simulink model "DTNS_KAISIM"  (R2022a)
settings: Solver=FixedStepDiscrete  StartTime=0.0  StopTime=200  FixedStep=0.04  RelTol=1e-3
PreLoadFcn:
  | listing = dir;
  | if (contains([listing .name], 'DTNS_KAISIM.slx'))
  |     addpath('./TCAF', './TRN', './FTG', './DYN', './FLCC', './GPS', './RALT', './INS', './MAP', './AGR');
  | else
  | 
  | end
  | 
  | load('BUS_STRUCTURE_DYN.mat');
  | load('BUS_STRUCTURE_FLCC.mat');
  | load('BUS_STRUCTURE_RALT.mat');
  | load('BUS_STRUCTURE_INS.mat');
  | load('BUS_STRUCTURE_GPS.mat');
  | load('BUS_STRUCTURE_SENSOR_INPUT.mat');
  | load('BusStructureTRN.mat');
  | load('BusStructureWTPG.mat');
  | load('BusStructureDTF.mat');
  | load('BusStructureGCAWS.mat');
  | load('BusStructureCR.mat');
  | load('BusStructureHR.mat');
  | load('BusStructureLOSR.mat');
  | 
  | clear logsout
InitFcn:
  | listing = dir;
  | if (contains([listing .name], 'DTNS_KAISIM.slx'))
  |     addpath('./TCAF', './TRN', './FTG', './DYN', './FLCC', './GPS', './RALT', './INS', './MAP', './AGR');
  | else
  | 
  | end
  | 
  | load('BUS_STRUCTURE_DYN.mat');
  | load('BUS_STRUCTURE_FLCC.mat');
  | load('BUS_STRUCTURE_RALT.mat');
  | load('BUS_STRUCTURE_INS.mat');
  | load('BUS_STRUCTURE_GPS.mat');
  | load('BUS_STRUCTURE_SENSOR_INPUT.mat');
  | load('BusStructureTRN.mat');
  | load('BusStructureWTPG.mat');
  | load('BusStructureDTF.mat');
  | load('BusStructureGCAWS.mat');
  | load('BusStructureCR.mat');
  | load('BusStructureHR.mat');
  | load('BusStructureLOSR.mat');
  | 
  | clear logsout
(part 1 of 2)
settings Model: Creator=ASCL  LastModifiedBy=halbu
settings SolverCC: PositivePriorityOrder=on
settings DataIOCC: ExternalInput=TCAF_WHOLESIMScenario.getElement('IN_TPF_WCPSIM_STICK'),TCAF_WHOLESIMScenario.getElement('IN_TPF_WCPSIM_FLIGHT_CMD'),TCAF_WHOLESIMScenario.getElement('IN_DTFIn'),TCAF_WHOLESIMScenario.getElement('IN_GCAWSIn')  SaveOutput=off  DSMLogging=off  ReturnWorkspaceOutputs=off
settings OptimizationCC: BlockReduction=off  DefaultParameterBehavior=Inlined  UseDivisionForNetSlopeComputation=on  GainParamInheritBuiltInType=on  UseFloatMulNetSlope=on  ExpressionFolding=off  PassReuseOutputArgsAs=Individual arguments  ZeroExternalMemoryAtStartup=off  ZeroInternalMemoryAtStartup=off  EfficientFloat2IntCast=on  LifeSpan=inf  OptimizeBlockOrder=speed  DifferentSizesBufferReuse=on  EfficientTunableParamExpr=on
settings DebuggingCC: SignalInfNanChecking=warning  ReadBeforeWriteMsg=EnableAllAsError  WriteAfterWriteMsg=EnableAllAsError  WriteAfterReadMsg=EnableAllAsError  IntegerOverflowMsg=error  ParameterTunabilityLossMsg=error  UniqueDataStoreMsg=error  AssertControl=DisableAll  NonBusSignalsTreatedAsBus=error  SFInvalidInputDataAccessInChartInitDiag=error  SFTransitionOutsideNaturalParentDiag=error  SFUnreachableExecutionPathDiag=error  SFUndirectedBroadcastEventsDiag=error  IntegerSaturationMsg=error
settings HardwareCC: ProdBitPerPointer=32  ProdBitPerSizeT=32  ProdBitPerPtrDiffT=32  ProdLargestAtomicInteger=Long  ProdLargestAtomicFloat=Double  ProdEndianess=BigEndian  ProdWordSize=32  ProdLongLongMode=on  ProdHWDeviceType=Freescale->MPC83xx
settings ModelReferenceCC: ModelReferenceNumInstancesAllowed=Single
settings SFSimCC: SimCustomHeaderCode="#include \"MAP.h\""  SimUserSources=MAP.c  SimUserLibraries=WS2_32.LIB  CompileTimeRecursionLimit=0  EnableRuntimeRecursion=off  MATLABDynamicMemAlloc=off
settings RTWCC: SystemTargetFile=ert.tlc  TemplateMakefile=ert_default_tmf  GenerateReport=on  RTWUseSimCustomCode=on  CustomHeaderCode="#include \"MAP.h\""  CustomSource=MAP.c  CustomLibrary=WS2_32.LIB  BuildConfiguration=Faster Runs  IncludeHyperlinkInReport=on  LaunchReport=on  GenerateTraceInfo=on  GenerateTraceReport=on  GenerateTraceReportSl=on  GenerateTraceReportSf=on  GenerateTraceReportEml=on
settings CodeAppCC: ForceParamTrailComments=on  IgnoreCustomStorageClasses=off  OperatorAnnotations=on  SimulinkDataObjDesc=on  SFDataObjDesc=on  MATLABFcnDesc=on  InsertBlockDesc=on  StateflowObjectComments=on  MATLABSourceComments=on  EnableCustomComments=on  InlinedPrmAccess=Macros  ReqsInCode=on
settings ERTTargetCC: TargetLangStandard=C99 (ISO)  UtilityFuncGeneration=Shared location  GenerateSampleERTMain=on  IncludeMdlTerminateFcn=off  CombineSignalStateStructs=on  SuppressErrorStatus=on  SupportAbsoluteTime=off  SupportNonFinite=off  SupportComplex=off  ParenthesesLevel=Standards  CastingMode=Standards  GenerateSharedConstants=off  InlinedParameterPlacement=NonHierarchical  ERTCustomFileTemplate=example_file_process.tlc  RateTransitionBlockCode=Function  PreserveIfCondition=on  ConvertIfToSwitch=off  EnableSignedLeftShifts=off  EnableSignedRightShifts=off

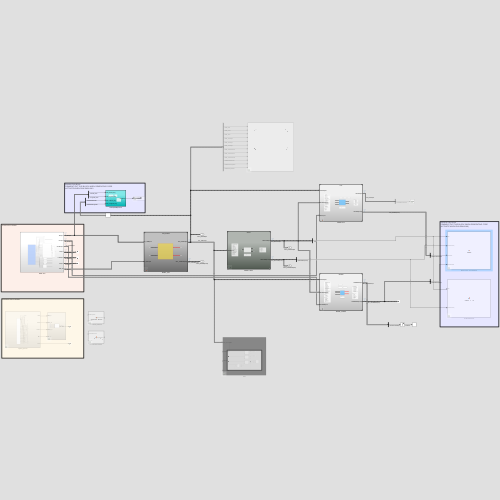
[thumbnail: Simulink's stored preview of the top-level diagram]
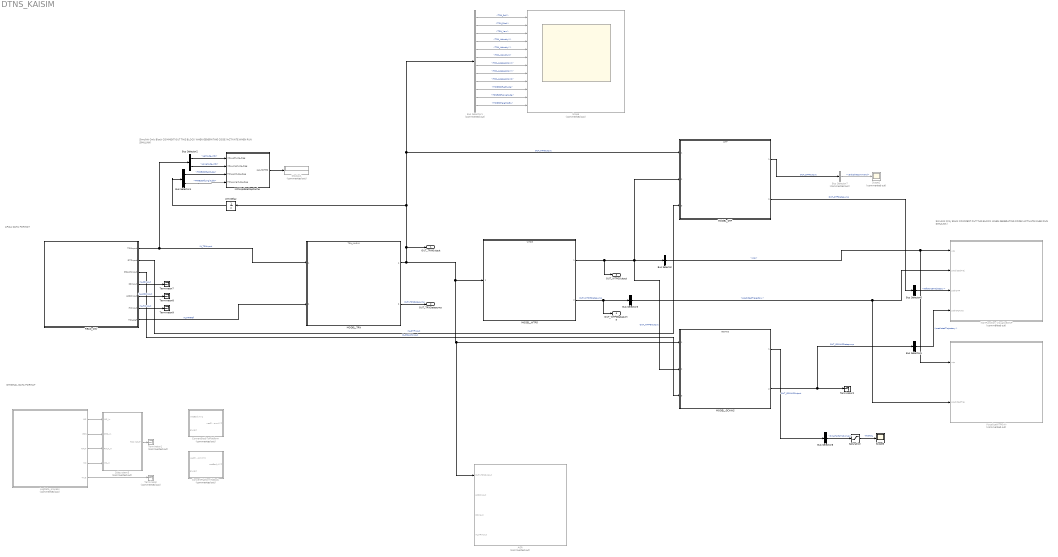
== system DTNS_KAISIM ==
  note: APIAA DATA FORMAT
  note: ORIGINAL DATA FORMAT
  note: Simulink Only Block
      | COMMENT OUT THIS BLOCK WHEN GENERATING CODE
      | (ACTIVATE WHEN RUN SIMULINK)
  note: Simulink Only Block
      | COMMENT OUT THIS BLOCK WHEN GENERATING CODE
      | (ACTIVATE WHEN RUN SIMULINK)
  AGR : Subsystem  Commented=on
  Bus Selector : BusSelector  OutputSignals=wtp
  Bus Selector1 : BusSelector  Commented=on  OutputSignals=TRN_Roll,TRN_Pitch,TRN_Yaw,TRN_VelocityX,TRN_VelocityY,TRN_VelocityZ,TRN_AccelerationX,TRN_AccelerationY,TRN_AccelerationZ,TRNEstOfLatitude,TRNEstOfLongitude,TRNEstHeightAGL
  Bus Selector2 : BusSelector  OutputSignals=Latitude_INS,Longitude_INS
  Bus Selector3 : BusSelector  OutputSignals=predictedTrajectory
  Bus Selector4 : BusSelector  OutputSignals=TRNEstOfLatitude,TRNEstOfLongitude
  Bus Selector5 : BusSelector  OutputSignals=predictedTrajectory
  Bus Selector6 : BusSelector  OutputSignals=referenceTrajectory
  Bus Selector7 : BusSelector  Commented=on  OutputSignals=verticalGCommand
  Bus Selector8 : BusSelector  OutputSignals=timeToGoToPullUp
  ConvertBodyToPlatform : MATLAB Function  Commented=on  TreatAsAtomicUnit=on
  ConvertPlatformToBody : MATLAB Function  Commented=on  TreatAsAtomicUnit=on
  Display1 : Display  Commented=on
  InitNUpdateMapCache : Subsystem  TreatAsAtomicUnit=on
  LogData_process : Subsystem  Commented=on
  MATFunction_VisualizeWCP : MATLAB Function  Commented=on  TreatAsAtomicUnit=on
  MODEL_DTF : ModelReference  ModelNameDialog=DTF.slx  SimulationMode=Normal  ModelReferenceVersion=1.428
  MODEL_GCAWS : ModelReference  ModelNameDialog=GCAWS.slx  SimulationMode=Normal  ModelReferenceVersion=1.774
  MODEL_TRN : ModelReference  ModelNameDialog=TRN_KAISIM.slx  SimulationMode=Normal  ModelReferenceVersion=2.352
  MODEL_WTPG : ModelReference  ModelNameDialog=WTPG.slx  SimulationMode=Normal  ModelReferenceVersion=1.377
  READ_CSV : Subsystem
  Saturation : Saturate  UpperLimit=5.0  LowerLimit=0.0
  Scope : Scope  Commented=on  NumInputPorts=12
  Scope1 : Scope  Commented=on
  Scope3 : Scope
  Subsystem3 : Subsystem  Commented=on
  Terminator : Terminator  Commented=on
  Terminator1 : Terminator  Commented=on
  Terminator{2,7..9} (4 alike) : Terminator
  Unit Delay : UnitDelay  SampleTime=-1  HasFrameUpgradeWarning=on
  VisualizeWTPOnly : MATLAB Function  Commented=on  TreatAsAtomicUnit=on
  OUT_TRNOutput : Outport  OutDataTypeStr=Bus: TRNOutput  BusOutputAsStruct=on
  OUT_TRNDatapump : Outport  Port=2  OutDataTypeStr=Bus: TRNDatapump
  OUT_WTPGOutput : Outport  Port=3  OutDataTypeStr=Bus: WTPGOutput
  OUT_WTPGDatapump : Outport  Port=4  OutDataTypeStr=Bus: WTPGDatapump
  wires:
  Bus Selector7/1 -> Scope1/1  "<verticalGCommand>"
  Bus Selector6/1 -> MATFunction_VisualizeWCP/3(pathDTF)  "<referenceTrajectory>"
  Bus Selector1/4 -> Scope/4  "<TRN_VelocityX>"
  MODEL_DTF/2 -> Bus Selector6/1  "OUT_DTFDatapump"
  Bus Selector5/1 -> MATFunction_VisualizeWCP/4(pathGCAWS)  "<predictedTrajectory>"
  Bus Selector1/5 -> Scope/5  "<TRN_VelocityY>"
  Bus Selector1/7 -> Scope/7  "<TRN_AccelerationX>"
  Bus Selector1/8 -> Scope/8  "<TRN_AccelerationY>"
  MODEL_WTPG/1 -> OUT_WTPGOutput/1, MODEL_GCAWS/2, MODEL_DTF/2, Bus Selector/1  "OUT_WTPGOutput"
  Bus Selector1/9 -> Scope/9  "<TRN_AccelerationZ>"
  Bus Selector1/12 -> Scope/12  "<TRNEstHeightAGL>"
  Bus Selector1/11 -> Scope/11  "<TRNEstOfLongitude>"
  MODEL_TRN/1 -> Unit Delay/1, Bus Selector1/1, MODEL_DTF/1, OUT_TRNOutput/1, AGR/1(OUT_TRNOutput), MODEL_GCAWS/1, MODEL_WTPG/1  "OUT_TRNOutput"
  MODEL_WTPG/2 -> OUT_WTPGDatapump/1, Bus Selector3/1  "OUT_WTPGDatapump"
  Bus Selector1/3 -> Scope/3  "<TRN_Yaw>"
  MODEL_GCAWS/2 -> Bus Selector5/1, Terminator2/1  "OUT_GCAWSDatapump"
  Bus Selector1/10 -> Scope/10  "<TRNEstOfLatitude>"
  MODEL_TRN/2 -> OUT_TRNDatapump/1  "OUT_TRNDatapump"
  MODEL_GCAWS/1 -> Bus Selector8/1  "OUT_GCAWSOutput"
  Bus Selector1/6 -> Scope/6  "<TRN_VelocityZ>"
  Bus Selector3/1 -> VisualizeWTPOnly/2(predictedTraj), MATFunction_VisualizeWCP/2(predictedTraj)  "<predictedTrajectory>"
  READ_CSV/1(TRNInput) -> Bus Selector2/1, MODEL_TRN/1  "IN_TRNInput"
  Bus Selector/1 -> VisualizeWTPOnly/1(wtp), MATFunction_VisualizeWCP/1(wtp)  "<wtp>"
  Bus Selector1/1 -> Scope/1  "<TRN_Roll>"
  MODEL_DTF/1 -> Bus Selector7/1  "OUT_DTFOutput"
  Bus Selector1/2 -> Scope/2  "<TRN_Pitch>"
  Bus Selector8/1 -> Saturation/1  "<timeToGoToPullUp>"
  Saturation/1 -> Scope3/1  "TTGTPU"
  READ_CSV/2(DTFInput) -> MODEL_DTF/3  "IN_DTFInput"
  READ_CSV/3(GCAWSInput) -> MODEL_GCAWS/3  "IN_GCAWSInput"
  Bus Selector2/1 -> InitNUpdateMapCache/1(INS_Latitude_Deg)  "<Latitude_INS>"
  Bus Selector2/2 -> InitNUpdateMapCache/2(INS_Longitude_Deg)  "<Longitude_INS>"
  READ_CSV/5(LOSRInput) -> Terminator8/1  "IN_LOSRInput"
  READ_CSV/4(CRInput) -> Terminator7/1  "IN_CRInput"
  InitNUpdateMapCache/1(resultDTED) -> Display1/1
  READ_CSV/6(HRInput) -> Terminator9/1  "IN_HRInput"
  LogData_process/1(INS) -> Subsystem3/1(INS_In)
  LogData_process/2(GPS) -> Subsystem3/2(GPS_In)
  LogData_process/3(RALT) -> Subsystem3/3(RALT_In)
  LogData_process/4(MC) -> Subsystem3/4(MC_In)
  LogData_process/5(True) -> Terminator/1
  Subsystem3/1(TRN INPUT) -> Terminator1/1
  READ_CSV/7(TRN_Ref) -> MODEL_TRN/2  "IN_TRNRef"
  Bus Selector4/1 -> InitNUpdateMapCache/3(TRN_Latitude_Deg)  "<TRNEstOfLatitude>"
  Bus Selector4/2 -> InitNUpdateMapCache/4(TRN_Longitude_Deg)  "<TRNEstOfLongitude>"
  Unit Delay/1 -> Bus Selector4/1

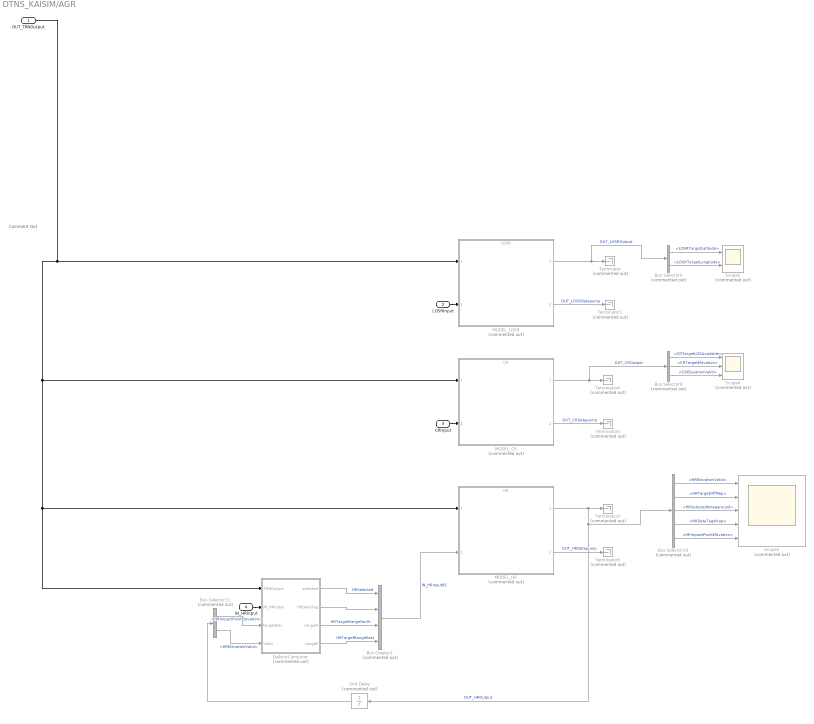
== system DTNS_KAISIM/AGR ==
  note: Comment Out
  OUT_TRNOutput : Inport
  LOSRInput : Inport  Port=2
  CRInput : Inport  Port=3
  IN_HRInput : Inport  Port=4
  BallisticComputer : MATLAB Function  Commented=on  TreatAsAtomicUnit=on
  Bus Creator3 : BusCreator  Commented=on  Inputs=4  OutDataTypeStr=Bus: HRInput  NonVirtualBus=on
      settings: InheritFromInputs=off
  Bus Selector10 : BusSelector  Commented=on  OutputSignals=HRElevationValid,HRTargetOffMap,HRSelectedWraparound,HRDataTagWrap,HRImpactPointElevation
  Bus Selector11 : BusSelector  Commented=on  OutputSignals=HRImpactPointElevation,HRElevationValid
  Bus Selector4 : BusSelector  Commented=on  OutputSignals=LOSRTargetLatitude,LOSRTargetLongitude
  Bus Selector9 : BusSelector  Commented=on  OutputSignals=CRTargetLOSAvailable,CRTargetElevation,CRElevationValid
  MODEL_CR : ModelReference  Commented=on  ModelNameDialog=CR.slx  SimulationMode=Normal  ModelReferenceVersion=1.236
  MODEL_HR : ModelReference  Commented=on  ModelNameDialog=HR.slx  SimulationMode=Normal  ModelReferenceVersion=1.371
  MODEL_LOSR : ModelReference  Commented=on  ModelNameDialog=LOSR.slx  SimulationMode=Normal  ModelReferenceVersion=1.331
  Scope2 : Scope  Commented=on  NumInputPorts=2
  Scope4 : Scope  Commented=on  NumInputPorts=3
  Scope5 : Scope  Commented=on  NumInputPorts=5
  Terminator{,1,3..6} (6 alike) : Terminator  Commented=on
  Unit Delay : UnitDelay  Commented=on  SampleTime=-1  HasFrameUpgradeWarning=on
  wires:
  MODEL_LOSR/1 -> Bus Selector4/1, Terminator/1  "OUT_LOSROutput"
  Bus Selector10/3 -> Scope5/3  "<HRSelectedWraparound>"
  MODEL_HR/1 -> Unit Delay/1, Bus Selector10/1, Terminator3/1  "OUT_HROutput"
  Bus Selector9/2 -> Scope4/2  "<CRTargetElevation>"
  BallisticComputer/2(HRDataTag) -> Bus Creator3/2
  Bus Creator3/1 -> MODEL_HR/2  "IN_HRInputBC"
  Bus Selector9/1 -> Scope4/1  "<CRTargetLOSAvailable>"
  MODEL_HR/2 -> Terminator6/1  "OUT_HRDatapump"
  Bus Selector10/1 -> Scope5/1  "<HRElevationValid>"
  MODEL_CR/1 -> Bus Selector9/1, Terminator4/1  "OUT_CROutput"
  Bus Selector4/2 -> Scope2/2  "<LOSRTargetLongitude>"
  OUT_TRNOutput/1 -> BallisticComputer/1(TRNOutput), MODEL_HR/1, MODEL_CR/1, MODEL_LOSR/1
  Bus Selector10/2 -> Scope5/2  "<HRTargetOffMap>"
  LOSRInput/1 -> MODEL_LOSR/2
  MODEL_CR/2 -> Terminator5/1  "OUT_CRDatapump"
  Bus Selector10/5 -> Scope5/5  "<HRImpactPointElevation>"
  MODEL_LOSR/2 -> Terminator1/1  "OUT_LOSRDatapump"
  BallisticComputer/4(rangeE) -> Bus Creator3/4  "HRTargetRangeEast"
  Bus Selector4/1 -> Scope2/1  "<LOSRTargetLatitude>"
  Bus Selector10/4 -> Scope5/4  "<HRDataTagWrap>"
  Unit Delay/1 -> Bus Selector11/1
  IN_HRInput/1 -> BallisticComputer/2(IN_HRInput)
  BallisticComputer/3(rangeN) -> Bus Creator3/3  "HRTargetRangeNorth"
  Bus Selector11/2 -> BallisticComputer/4(Valid)  "<HRElevationValid>"
  Bus Selector9/3 -> Scope4/3  "<CRElevationValid>"
  BallisticComputer/1(selected) -> Bus Creator3/1  "HRSelected"
  Bus Selector11/1 -> BallisticComputer/3(targetElev)  "<HRImpactPointElevation>"
  CRInput/1 -> MODEL_CR/2

== system DTNS_KAISIM/InitNUpdateMapCache ==
  INS_Latitude_Deg : Inport  OutDataTypeStr=double
  INS_Longitude_Deg : Inport  Port=2  OutDataTypeStr=double
  TRN_Latitude_Deg : Inport  Port=3
  TRN_Longitude_Deg : Inport  Port=4
  If : If  NumInputs=2  IfExpression=(u1 == 0)  ShowElse=off
  InitializeMAP : MATLAB Function  TreatAsAtomicUnit=on
  UpdateCache : Subsystem  TreatAsAtomicUnit=on
  resultDTED : Outport  VectorParamsAs1DForOutWhenUnconnected=off
  wires:
  INS_Longitude_Deg/1 -> UpdateCache/2(INS_Longitude_Deg)
  UpdateCache/1(result) -> resultDTED/1
  InitializeMAP/1(successDTED) -> If/1
  INS_Latitude_Deg/1 -> UpdateCache/1(INS_Latitude_Deg)
  InitializeMAP/2(successDVOF) -> If/2
  If/1 -> UpdateCache/Action
  TRN_Latitude_Deg/1 -> UpdateCache/3(TRN_Latitude_Deg)
  TRN_Longitude_Deg/1 -> UpdateCache/4(TRN_Longitude_Deg)

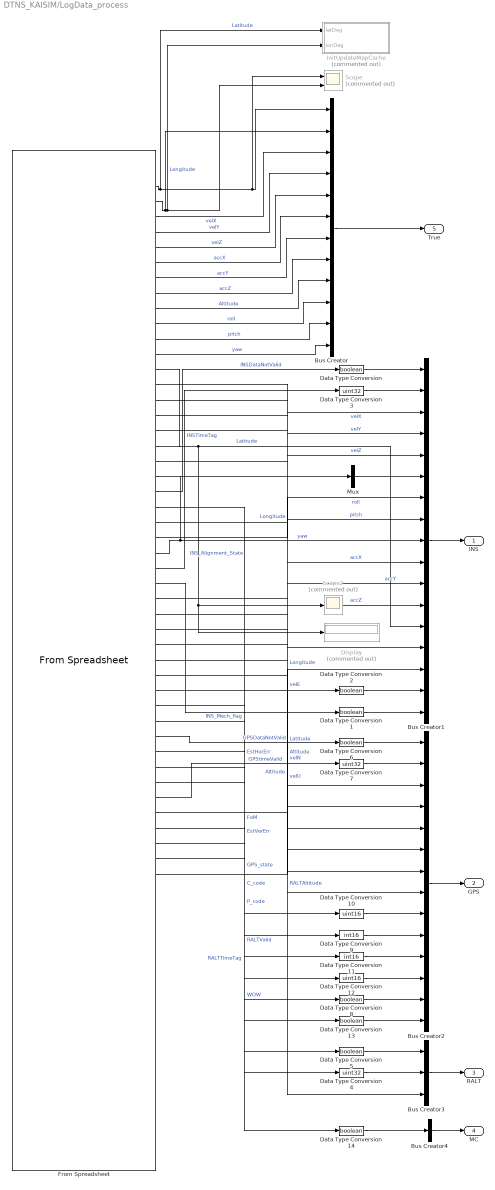
== system DTNS_KAISIM/LogData_process ==
  Bus Creator : BusCreator  Inputs=12  OutDataTypeStr=Bus: TRN_Ref
      settings: InheritFromInputs=off
  Bus Creator1 : BusCreator  Inputs=17  OutDataTypeStr=Bus: TRN_INS
      settings: InheritFromInputs=off
  Bus Creator2 : BusCreator  Inputs=14  OutDataTypeStr=Bus: TRN_GPS
      settings: InheritFromInputs=off
  Bus Creator3 : BusCreator  Inputs=3  OutDataTypeStr=Bus: TRN_RALT
      settings: InheritFromInputs=off
  Bus Creator4 : BusCreator  Inputs=1  OutDataTypeStr=Bus: TRN_MC
      settings: InheritFromInputs=off
  Data Type Conversion{,1..2,5..6,8,13..14} (8 alike) : DataTypeConversion  OutDataTypeStr=boolean  SaturateOnIntegerOverflow=off  RndMeth=Floor
  Data Type Conversion10 : DataTypeConversion  OutDataTypeStr=uint16  SaturateOnIntegerOverflow=off  RndMeth=Floor
  Data Type Conversion11 : DataTypeConversion  OutDataTypeStr=int16  SaturateOnIntegerOverflow=off  RndMeth=Floor
  Data Type Conversion12 : DataTypeConversion  OutDataTypeStr=uint16  SaturateOnIntegerOverflow=off  RndMeth=Floor
  Data Type Conversion3 : DataTypeConversion  OutDataTypeStr=uint32  SaturateOnIntegerOverflow=off  RndMeth=Floor
  Data Type Conversion4 : DataTypeConversion  OutDataTypeStr=uint32  SaturateOnIntegerOverflow=off  RndMeth=Floor
  Data Type Conversion7 : DataTypeConversion  OutDataTypeStr=uint32  SaturateOnIntegerOverflow=off  RndMeth=Floor
  Data Type Conversion9 : DataTypeConversion  OutDataTypeStr=int16  SaturateOnIntegerOverflow=off  RndMeth=Floor
  Display : Display  Commented=on
  From Spreadsheet : FromSpreadsheet  FileName=KAI_input.csv  SheetName=KAI_input  TreatFirstColumnAs=Data  SampleTime=-1
  InitUpdateMapCache : Subsystem  Commented=on  TreatAsAtomicUnit=on
  Mux : Mux  Inputs=1
  Scope : Scope  Commented=on  NumInputPorts=2
  Scope2 : Scope  Commented=on
  INS : Outport  OutDataTypeStr=Bus: TRN_INS
  GPS : Outport  Port=2  OutDataTypeStr=Bus: TRN_GPS
  RALT : Outport  Port=3  OutDataTypeStr=Bus: TRN_RALT
  MC : Outport  Port=4  OutDataTypeStr=Bus: TRN_MC
  True : Outport  Port=5  OutDataTypeStr=Bus: TRN_Ref
  wires:
  From Spreadsheet/23 -> Data Type Conversion2/1  "INS_Alignment_State"
  From Spreadsheet/22 -> Data Type Conversion/1  "INSDataNotValid"
  From Spreadsheet/21 -> Bus Creator1/12  "accZ"
  From Spreadsheet/20 -> Bus Creator1/11  "accY"
  Bus Creator/1 -> True/1
  From Spreadsheet/27 -> Data Type Conversion3/1  "INSTimeTag"
  From Spreadsheet/25 -> Bus Creator1/8  "pitch"
  From Spreadsheet/24 -> Bus Creator1/7  "roll"
  From Spreadsheet/4 -> Bus Creator/3  "velX"
  From Spreadsheet/5 -> Bus Creator/4  "velY"
  From Spreadsheet/6 -> Bus Creator/5  "velZ"
  From Spreadsheet/7 -> Bus Creator/6  "accX"
  From Spreadsheet/8 -> Bus Creator/7  "accY"
  From Spreadsheet/9 -> Bus Creator/8  "accZ"
  From Spreadsheet/10 -> Bus Creator/9  "Altitude"
  From Spreadsheet/11 -> Bus Creator/10  "roll"
  From Spreadsheet/12 -> Bus Creator/11  "pitch"
  From Spreadsheet/13 -> Bus Creator/12  "yaw"
  From Spreadsheet/15 -> Bus Creator1/14  "Longitude"
  From Spreadsheet/19 -> Bus Creator1/10  "accX"
  From Spreadsheet/16 -> Bus Creator1/3  "velX"
  From Spreadsheet/17 -> Bus Creator1/4  "velY"
  From Spreadsheet/18 -> Bus Creator1/5  "velZ"
  Bus Creator1/1 -> INS/1
  From Spreadsheet/36 -> Data Type Conversion11/1  "EstVerErr"
  From Spreadsheet/37 -> Data Type Conversion10/1  "FoM"
  From Spreadsheet/38 -> Data Type Conversion6/1  "GPSDataNotValid"
  From Spreadsheet/39 -> Data Type Conversion12/1  "GPS_state"
  Bus Creator3/1 -> RALT/1
  Bus Creator2/1 -> GPS/1
  From Spreadsheet/28 -> Data Type Conversion1/1  "INS_Mech_flag"
  From Spreadsheet/29 -> Bus Creator2/3  "Latitude"
  From Spreadsheet/30 -> Bus Creator2/4  "Longitude"
  From Spreadsheet/31 -> Bus Creator2/6  "velE"
  From Spreadsheet/34 -> Bus Creator2/5  "Altitude"
  From Spreadsheet/35 -> Data Type Conversion9/1  "EstHorErr"
  From Spreadsheet/33 -> Bus Creator2/8  "velU"
  From Spreadsheet/32 -> Bus Creator2/7  "velN"
  Bus Creator4/1 -> MC/1
  Data Type Conversion/1 -> Bus Creator1/1
  Data Type Conversion3/1 -> Bus Creator1/2
  Data Type Conversion2/1 -> Bus Creator1/16
  Data Type Conversion5/1 -> Bus Creator3/1
  Data Type Conversion4/1 -> Bus Creator3/2
  Data Type Conversion7/1 -> Bus Creator2/2
  Data Type Conversion6/1 -> Bus Creator2/1
  Data Type Conversion1/1 -> Bus Creator1/17
  Data Type Conversion10/1 -> Bus Creator2/9
  Data Type Conversion8/1 -> Bus Creator2/13
  Data Type Conversion9/1 -> Bus Creator2/10
  From Spreadsheet/46 -> Data Type Conversion14/1  "WOW"
  From Spreadsheet/45 -> Data Type Conversion4/1  "RALTTimeTag"
  From Spreadsheet/44 -> Data Type Conversion5/1  "RALTValid"
  From Spreadsheet/47 -> Bus Creator1/15  "Altitude"
  Data Type Conversion14/1 -> Bus Creator4/1
  Data Type Conversion13/1 -> Bus Creator2/14
  From Spreadsheet/40 -> Data Type Conversion8/1  "C_code"
  From Spreadsheet/41 -> Data Type Conversion13/1  "P_code"
  From Spreadsheet/42 -> Data Type Conversion7/1  "GPStimeValid"
  From Spreadsheet/43 -> Bus Creator3/3  "RALTAltitude"
  Data Type Conversion12/1 -> Bus Creator2/12
  Data Type Conversion11/1 -> Bus Creator2/11
  Mux/1 -> Bus Creator1/6
  From Spreadsheet/2 -> Scope/1, Bus Creator/1, InitUpdateMapCache/1(latDeg)  "Latitude"
  From Spreadsheet/3 -> InitUpdateMapCache/2(lonDeg), Scope/2, Bus Creator/2  "Longitude"
  From Spreadsheet/26 -> Mux/1, Bus Creator1/9  "yaw"
  From Spreadsheet/14 -> Display/1, Scope2/1, Bus Creator1/13  "Latitude"

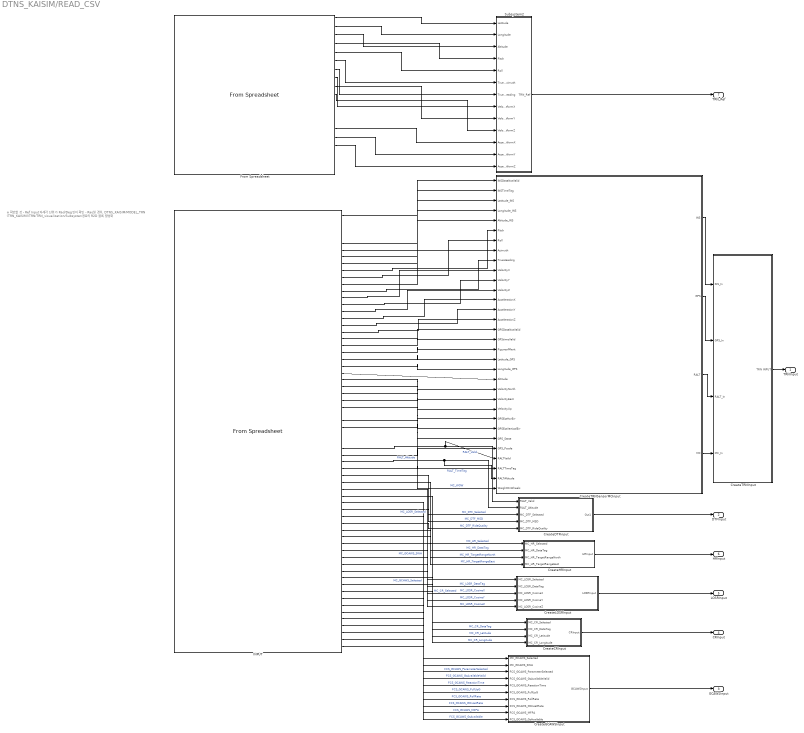
== system DTNS_KAISIM/READ_CSV ==
  note: ※ 확인할 것
      | - Ref Input 자세각 단위가 Rad/Deg 인지 확인
      | - Rad일 경우, DTNS_KAISIM/MODEL_TRN (TRN_KAISIM)/TRN/TRN_visualization/Subsystem2 경로의 R2D 블록 활성화
  CreateCRInput : Subsystem
  CreateDTFInput : Subsystem
  CreateGCAWSInput : Subsystem
  CreateHRInput : Subsystem
  CreateLOSRInput : Subsystem
  CreateTRNInput : Subsystem
  CreateTRNSensorMCInput : Subsystem
  From Spreadsheet : FromSpreadsheet  FileName=C:\Users\halbu\Documents\GitHub\DTNS\data\test_TRUE.csv  SheetName=test_TRUE  OutDataTypeStr=double  SampleTime=0.04  ExtrapolationBeforeFirstDataPoint=Hold first value  InterpolationWithinTimeRange=Zero order hold  ExtrapolationAfterLastDataPoint=Hold last value
  INPUT : FromSpreadsheet  FileName=C:\Users\halbu\Documents\GitHub\DTNS\data\test_INPUT.csv  SheetName=test_INPUT  OutDataTypeStr=double  SampleTime=0.04  ExtrapolationBeforeFirstDataPoint=Hold first value  InterpolationWithinTimeRange=Zero order hold  ExtrapolationAfterLastDataPoint=Hold last value
  Subsystem2 : Subsystem
  TRNInput : Outport  OutDataTypeStr=Bus: TRNInput
  DTFInput : Outport  Port=2  OutDataTypeStr=Bus: DTFInput
  GCAWSInput : Outport  Port=3  OutDataTypeStr=Bus: GCAWSInput
  CRInput : Outport  Port=4  OutDataTypeStr=Bus: CRInput
  LOSRInput : Outport  Port=5  OutDataTypeStr=Bus: LOSRInput
  HRInput : Outport  Port=6  OutDataTypeStr=Bus: HRInput
  TRN_Ref : Outport  Port=7  OutDataTypeStr=Bus: TRN_Ref
  wires:
  Subsystem2/1(TRN_Ref) -> TRN_Ref/1
  INPUT/7 -> CreateTRNSensorMCInput/4(Longitude_INS)
  INPUT/6 -> CreateTRNSensorMCInput/3(Latitude_INS)
  INPUT/5 -> CreateTRNSensorMCInput/2(INSTimeTag)
  INPUT/14 -> CreateTRNSensorMCInput/11(VelocityY)
  INPUT/10 -> CreateTRNSensorMCInput/7(Roll)
  INPUT/22 -> CreateTRNSensorMCInput/19(Latitude_GPS)
  INPUT/11 -> CreateTRNSensorMCInput/8(Azimuth)
  INPUT/23 -> CreateTRNSensorMCInput/20(Longitude_GPS)
  INPUT/19 -> CreateTRNSensorMCInput/16(GPSDataNotValid)
  INPUT/13 -> CreateTRNSensorMCInput/10(VelocityX)
  INPUT/9 -> CreateTRNSensorMCInput/6(Pitch)
  INPUT/17 -> CreateTRNSensorMCInput/14(AccelerationY)
  CreateTRNSensorMCInput/2(GPS) -> CreateTRNInput/2(GPS_In)
  INPUT/21 -> CreateTRNSensorMCInput/18(FigureofMerit)
  CreateTRNSensorMCInput/1(INS) -> CreateTRNInput/1(INS_In)
  INPUT/57 -> CreateGCAWSInput/3(FCS_GCAWS_ParameterSelected)  "FCS_GCAWS_ParameterSelected"
  INPUT/61 -> CreateGCAWSInput/7(FCS_GCAWS_RollRate)  "FCS_GCAWS_RollRate"
  INPUT/58 -> CreateGCAWSInput/4(FCS_GCAWS_GsAvailableValid)  "FCS_GCAWS_GsAvailableValid"
  INPUT/62 -> CreateGCAWSInput/8(FCS_GCAWS_GOnsetRate)  "FCS_GCAWS_GOnsetRate"
  INPUT/59 -> CreateGCAWSInput/5(FCS_GCAWS_ReactionTime)  "FCS_GCAWS_ReactionTime"
  INPUT/63 -> CreateGCAWSInput/9(FCS_GCAWS_MFPA)  "FCS_GCAWS_MFPA"
  CreateGCAWSInput/1(GCAWSInput) -> GCAWSInput/1
  INPUT/60 -> CreateGCAWSInput/6(FCS_GCAWS_PullUpG)  "FCS_GCAWS_PullUpG"
  INPUT/64 -> CreateGCAWSInput/10(FCS_GCAWS_GsAvailable)  "FCS_GCAWS_GsAvailable"
  INPUT/56 -> CreateCRInput/4(MC_CR_Longitude)  "MC_CR_Longitude"
  CreateCRInput/1(CRInput) -> CRInput/1
  CreateLOSRInput/1(LOSRInput) -> LOSRInput/1
  INPUT/43 -> CreateGCAWSInput/1(MC_GCAWS_Selected)  "MC_GCAWS_Selected"
  INPUT/55 -> CreateCRInput/3(MC_CR_Latitude)  "MC_CR_Latitude"
  INPUT/51 -> CreateLOSRInput/3(MC_LOSR_CosineX)  "MC_LOSR_CosineX"
  INPUT/47 -> CreateHRInput/2(MC_HR_DataTag)  "MC_HR_DataTag"
  INPUT/45 -> CreateGCAWSInput/2(MC_GCAWS_SWH)  "MC_GCAWS_SWH"
  INPUT/41 -> CreateLOSRInput/1(MC_LOSR_Selected)  "MC_LOSR_Selected"
  INPUT/53 -> CreateLOSRInput/5(MC_LOSR_CosineZ)  "MC_LOSR_CosineZ"
  INPUT/49 -> CreateHRInput/4(MC_HR_TargetRangeEast)  "MC_HR_TargetRangeEast"
  CreateHRInput/1(HRInput) -> HRInput/1
  INPUT/52 -> CreateLOSRInput/4(MC_LOSR_CosineY)  "MC_LOSR_CosineY"
  INPUT/40 -> CreateHRInput/1(MC_HR_Selected)  "MC_HR_Selected"
  INPUT/48 -> CreateHRInput/3(MC_HR_TargetRangeNorth)  "MC_HR_TargetRangeNorth"
  INPUT/44 -> CreateDTFInput/4(MC_DTF_MSD)  "MC_DTF_MSD"
  INPUT/42 -> CreateCRInput/1(MC_CR_Selected)  "MC_CR_Selected"
  INPUT/54 -> CreateCRInput/2(MC_CR_DataTag)  "MC_CR_DataTag"
  INPUT/50 -> CreateLOSRInput/2(MC_LOSR_DataTag)  "MC_LOSR_DataTag"
  INPUT/46 -> CreateDTFInput/5(MC_DTF_RideQuality)  "MC_DTF_RideQuality"
  CreateDTFInput/1(Out1) -> DTFInput/1
  INPUT/8 -> CreateTRNSensorMCInput/5(Altitude_INS)
  INPUT/20 -> CreateTRNSensorMCInput/17(GPStimeValid)
  CreateTRNInput/1(TRN INPUT) -> TRNInput/1
  INPUT/1 -> CreateTRNSensorMCInput/1(INSDataNotValid)
  INPUT/26 -> CreateTRNSensorMCInput/23(VelocityEast)
  INPUT/38 -> CreateTRNSensorMCInput/32(WeightOnWheels)  "MC_WOW"
  INPUT/37 -> CreateTRNSensorMCInput/31(RALTAltitude), CreateDTFInput/2(RALT_Altitude)  "RALT_Altitude"
  INPUT/25 -> CreateTRNSensorMCInput/22(VelocityNorth)
  INPUT/29 -> CreateTRNSensorMCInput/26(GPSEstVerticalErr)
  INPUT/24 -> CreateTRNSensorMCInput/21(Altitude)
  INPUT/32 -> CreateTRNSensorMCInput/27(GPS_State)
  INPUT/36 -> CreateTRNSensorMCInput/30(RALTTimeTag)  "RALT_TimeTag"
  INPUT/28 -> CreateTRNSensorMCInput/25(GPSEstHorErr)
  INPUT/35 -> CreateTRNSensorMCInput/29(RALTValid), CreateDTFInput/1(RALT_Valid)  "RALT_Valid"
  INPUT/39 -> CreateDTFInput/3(MC_DTF_Selected)  "MC_DTF_Selected"
  INPUT/31 -> CreateTRNSensorMCInput/28(GPS_Pcode)
  INPUT/27 -> CreateTRNSensorMCInput/24(VelocityUp)
  INPUT/15 -> CreateTRNSensorMCInput/12(VelocityZ)
  INPUT/18 -> CreateTRNSensorMCInput/15(AccelerationZ)
  INPUT/12 -> CreateTRNSensorMCInput/9(TrueHeading)
  INPUT/16 -> CreateTRNSensorMCInput/13(AccelerationX)
  CreateTRNSensorMCInput/3(RALT) -> CreateTRNInput/3(RALT_In)
  CreateTRNSensorMCInput/4(MC) -> CreateTRNInput/4(MC_In)
  From Spreadsheet/1 -> Subsystem2/1(Latitude)
  From Spreadsheet/2 -> Subsystem2/2(Longitude)
  From Spreadsheet/3 -> Subsystem2/3(Altitude)
  From Spreadsheet/4 -> Subsystem2/4(Pitch)
  From Spreadsheet/5 -> Subsystem2/5(Roll)
  From Spreadsheet/7 -> Subsystem2/7(TrueHeading)
  From Spreadsheet/8 -> Subsystem2/8(VelocityPlatformX)
  From Spreadsheet/6 -> Subsystem2/6(TrueAzimuth)
  From Spreadsheet/14 -> Subsystem2/11(AccelerationPlatformX)
  From Spreadsheet/15 -> Subsystem2/12(AccelerationPlatformY)
  From Spreadsheet/16 -> Subsystem2/13(AccelerationPlatformZ)
  From Spreadsheet/9 -> Subsystem2/9(VelocityPlatformY)
  From Spreadsheet/10 -> Subsystem2/10(VelocityPlatformZ)

== system DTNS_KAISIM/Subsystem3 ==
  INS_In : Inport  OutDataTypeStr=Bus: TRN_INS
  GPS_In : Inport  Port=2  OutDataTypeStr=Bus: TRN_GPS
  RALT_In : Inport  Port=3  OutDataTypeStr=Bus: TRN_RALT
  MC_In : Inport  Port=4  OutDataTypeStr=Bus: TRN_MC
  Dataprocess1 : Subsystem
  TRN INPUT : Outport  OutDataTypeStr=Bus: TRNInput  VectorParamsAs1DForOutWhenUnconnected=off
  wires:
  GPS_In/1 -> Dataprocess1/1(In_GPS)
  Dataprocess1/1(TRN INPUT) -> TRN INPUT/1
  RALT_In/1 -> Dataprocess1/3(In_RALT)
  MC_In/1 -> Dataprocess1/4(IN_MC)
  INS_In/1 -> Dataprocess1/2(In_INS)

== system DTNS_KAISIM/InitNUpdateMapCache/UpdateCache ==
  INS_Latitude_Deg : Inport
  INS_Longitude_Deg : Inport  Port=2
  TRN_Latitude_Deg : Inport  Port=3
  TRN_Longitude_Deg : Inport  Port=4
  Action Port : ActionPort  ActionPortLabel=if((u1 == 0))
  UpdateCache : MATLAB Function  TreatAsAtomicUnit=on
  result : Outport  VectorParamsAs1DForOutWhenUnconnected=off
  wires:
  UpdateCache/1(result) -> result/1
  TRN_Latitude_Deg/1 -> UpdateCache/3(TRN_Latitude_Deg)
  TRN_Longitude_Deg/1 -> UpdateCache/4(TRN_Longitude_Deg)
  INS_Latitude_Deg/1 -> UpdateCache/1(INS_Latitude_Deg)
  INS_Longitude_Deg/1 -> UpdateCache/2(INS_Longitude_Deg)

== system DTNS_KAISIM/LogData_process/InitUpdateMapCache ==
  latDeg : Inport  OutDataTypeStr=double
  lonDeg : Inport  Port=2  OutDataTypeStr=double
  Caching : Subsystem  TreatAsAtomicUnit=on
  If1 : If  NumInputs=2  IfExpression=(u1 == 0)  ShowElse=off
  InitializeMAP : MATLAB Function  TreatAsAtomicUnit=on
  Scope : Scope
  Scope2 : Scope  NumInputPorts=2
  wires:
  lonDeg/1 -> Caching/2(lon)
  InitializeMAP/1(successDTED) -> If1/1, Scope2/1
  latDeg/1 -> Scope/1, Caching/1(lat)
  InitializeMAP/2(successDVOF) -> If1/2, Scope2/2
  If1/1 -> Caching/Action

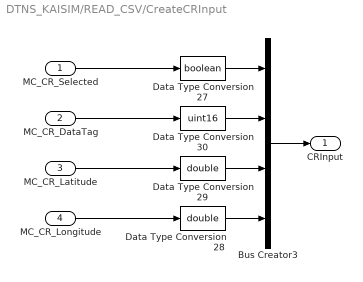
== system DTNS_KAISIM/READ_CSV/CreateCRInput ==
  MC_CR_Selected : Inport
  MC_CR_DataTag : Inport  Port=2
  MC_CR_Latitude : Inport  Port=3
  MC_CR_Longitude : Inport  Port=4
  Bus Creator3 : BusCreator  Inputs=4  OutDataTypeStr=Bus: CRInput  NonVirtualBus=on
      settings: InheritFromInputs=off
  Data Type Conversion27 : DataTypeConversion  OutDataTypeStr=boolean  RndMeth=Nearest  SaturateOnIntegerOverflow=off
  Data Type Conversion28 : DataTypeConversion  OutDataTypeStr=double  RndMeth=Nearest  SaturateOnIntegerOverflow=off
  Data Type Conversion29 : DataTypeConversion  OutDataTypeStr=double  RndMeth=Nearest  SaturateOnIntegerOverflow=off
  Data Type Conversion30 : DataTypeConversion  OutDataTypeStr=uint16  RndMeth=Nearest  SaturateOnIntegerOverflow=off
  CRInput : Outport
  wires:
  Data Type Conversion28/1 -> Bus Creator3/4
  MC_CR_Latitude/1 -> Data Type Conversion29/1
  Data Type Conversion27/1 -> Bus Creator3/1
  Data Type Conversion29/1 -> Bus Creator3/3
  Bus Creator3/1 -> CRInput/1
  Data Type Conversion30/1 -> Bus Creator3/2
  MC_CR_Longitude/1 -> Data Type Conversion28/1
  MC_CR_DataTag/1 -> Data Type Conversion30/1
  MC_CR_Selected/1 -> Data Type Conversion27/1

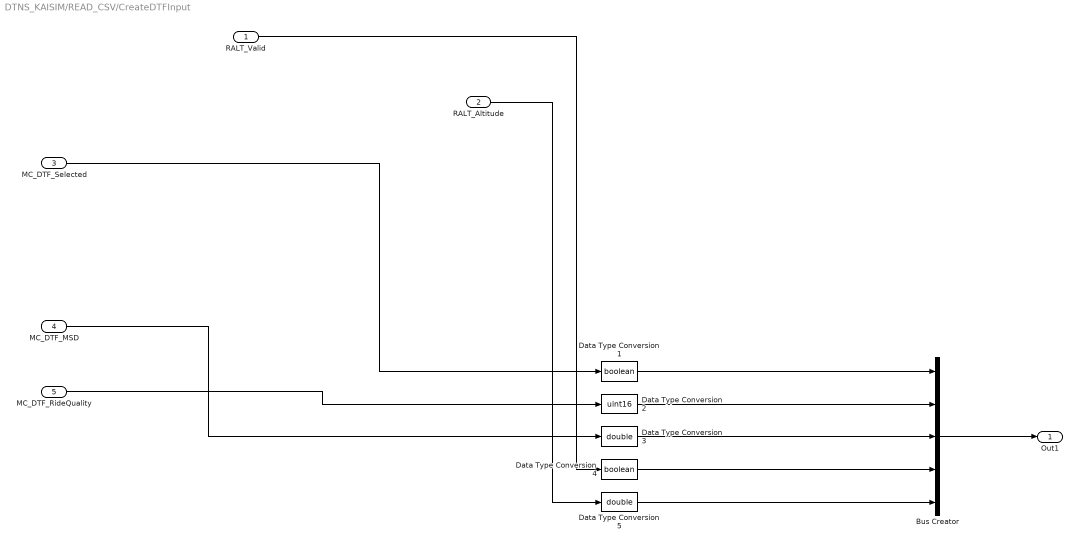
== system DTNS_KAISIM/READ_CSV/CreateDTFInput ==
  RALT_Valid : Inport
  RALT_Altitude : Inport  Port=2
  MC_DTF_Selected : Inport  Port=3
  MC_DTF_MSD : Inport  Port=4
  MC_DTF_RideQuality : Inport  Port=5
  Bus Creator : BusCreator  Inputs=5  OutDataTypeStr=Bus: DTFInput  NonVirtualBus=on
      settings: InheritFromInputs=off
  Data Type Conversion1 : DataTypeConversion  OutDataTypeStr=boolean  RndMeth=Nearest  SaturateOnIntegerOverflow=off
  Data Type Conversion2 : DataTypeConversion  OutDataTypeStr=uint16  RndMeth=Nearest  SaturateOnIntegerOverflow=off
  Data Type Conversion3 : DataTypeConversion  OutDataTypeStr=double  RndMeth=Nearest  SaturateOnIntegerOverflow=off
  Data Type Conversion4 : DataTypeConversion  OutDataTypeStr=boolean  RndMeth=Nearest  SaturateOnIntegerOverflow=off
  Data Type Conversion5 : DataTypeConversion  OutDataTypeStr=double  RndMeth=Nearest  SaturateOnIntegerOverflow=off
  Out1 : Outport
  wires:
  Data Type Conversion5/1 -> Bus Creator/5
  RALT_Altitude/1 -> Data Type Conversion5/1
  Data Type Conversion3/1 -> Bus Creator/3
  Bus Creator/1 -> Out1/1
  Data Type Conversion2/1 -> Bus Creator/2
  Data Type Conversion4/1 -> Bus Creator/4
  Data Type Conversion1/1 -> Bus Creator/1
  RALT_Valid/1 -> Data Type Conversion4/1
  MC_DTF_Selected/1 -> Data Type Conversion1/1
  MC_DTF_RideQuality/1 -> Data Type Conversion2/1
  MC_DTF_MSD/1 -> Data Type Conversion3/1

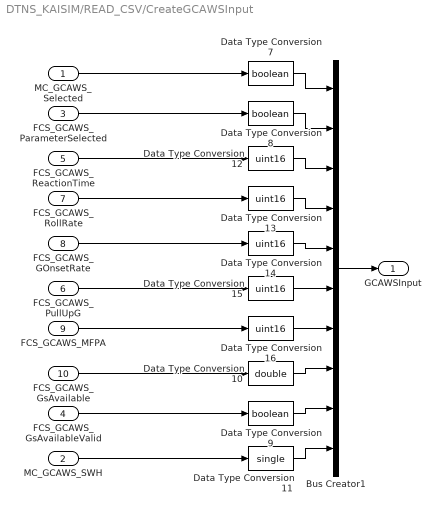
== system DTNS_KAISIM/READ_CSV/CreateGCAWSInput ==
  MC_GCAWS_Selected : Inport
  MC_GCAWS_SWH : Inport  Port=2
  FCS_GCAWS_ParameterSelected : Inport  Port=3
  FCS_GCAWS_GsAvailableValid : Inport  Port=4
  FCS_GCAWS_ReactionTime : Inport  Port=5
  FCS_GCAWS_PullUpG : Inport  Port=6
  FCS_GCAWS_RollRate : Inport  Port=7
  FCS_GCAWS_GOnsetRate : Inport  Port=8
  FCS_GCAWS_MFPA : Inport  Port=9
  FCS_GCAWS_GsAvailable : Inport  Port=10
  Bus Creator1 : BusCreator  Inputs=10  OutDataTypeStr=Bus: GCAWSInput  NonVirtualBus=on
      settings: InheritFromInputs=off
  Data Type Conversion10 : DataTypeConversion  OutDataTypeStr=double  RndMeth=Nearest  SaturateOnIntegerOverflow=off
  Data Type Conversion11 : DataTypeConversion  OutDataTypeStr=single  RndMeth=Nearest  SaturateOnIntegerOverflow=off
  Data Type Conversion{12..16} (5 alike) : DataTypeConversion  OutDataTypeStr=uint16  RndMeth=Nearest  SaturateOnIntegerOverflow=off
  Data Type Conversion7 : DataTypeConversion  OutDataTypeStr=boolean  RndMeth=Nearest  SaturateOnIntegerOverflow=off
  Data Type Conversion8 : DataTypeConversion  OutDataTypeStr=boolean  RndMeth=Nearest  SaturateOnIntegerOverflow=off
  Data Type Conversion9 : DataTypeConversion  OutDataTypeStr=boolean  RndMeth=Nearest  SaturateOnIntegerOverflow=off
  GCAWSInput : Outport
  wires:
  FCS_GCAWS_ReactionTime/1 -> Data Type Conversion12/1
  Data Type Conversion7/1 -> Bus Creator1/1
  Bus Creator1/1 -> GCAWSInput/1
  MC_GCAWS_SWH/1 -> Data Type Conversion11/1
  FCS_GCAWS_ParameterSelected/1 -> Data Type Conversion8/1
  FCS_GCAWS_RollRate/1 -> Data Type Conversion13/1
  FCS_GCAWS_PullUpG/1 -> Data Type Conversion15/1
  FCS_GCAWS_GOnsetRate/1 -> Data Type Conversion14/1
  FCS_GCAWS_MFPA/1 -> Data Type Conversion16/1
  Data Type Conversion13/1 -> Bus Creator1/4
  Data Type Conversion12/1 -> Bus Creator1/3
  Data Type Conversion8/1 -> Bus Creator1/2
  Data Type Conversion9/1 -> Bus Creator1/9
  Data Type Conversion15/1 -> Bus Creator1/6
  FCS_GCAWS_GsAvailable/1 -> Data Type Conversion10/1
  MC_GCAWS_Selected/1 -> Data Type Conversion7/1
  Data Type Conversion14/1 -> Bus Creator1/5
  Data Type Conversion10/1 -> Bus Creator1/8
  FCS_GCAWS_GsAvailableValid/1 -> Data Type Conversion9/1
  Data Type Conversion16/1 -> Bus Creator1/7
  Data Type Conversion11/1 -> Bus Creator1/10

== system DTNS_KAISIM/READ_CSV/CreateHRInput ==
  MC_HR_Selected : Inport
  MC_HR_DataTag : Inport  Port=2
  MC_HR_TargetRangeNorth : Inport  Port=3
  MC_HR_TargetRangeEast : Inport  Port=4
  Bus Creator5 : BusCreator  Inputs=4  OutDataTypeStr=Bus: HRInput  NonVirtualBus=on
      settings: InheritFromInputs=off
  Data Type Conversion36 : DataTypeConversion  OutDataTypeStr=boolean  RndMeth=Nearest  SaturateOnIntegerOverflow=off
  Data Type Conversion37 : DataTypeConversion  OutDataTypeStr=uint16  RndMeth=Nearest  SaturateOnIntegerOverflow=off
  Data Type Conversion38 : DataTypeConversion  OutDataTypeStr=double  RndMeth=Nearest  SaturateOnIntegerOverflow=off
  Data Type Conversion39 : DataTypeConversion  OutDataTypeStr=double  RndMeth=Nearest  SaturateOnIntegerOverflow=off
  HRInput : Outport  OutDataTypeStr=Bus: HRInput
  wires:
  MC_HR_Selected/1 -> Data Type Conversion36/1
  Data Type Conversion37/1 -> Bus Creator5/2
  Data Type Conversion39/1 -> Bus Creator5/4
  Data Type Conversion38/1 -> Bus Creator5/3
  MC_HR_TargetRangeNorth/1 -> Data Type Conversion38/1
  MC_HR_TargetRangeEast/1 -> Data Type Conversion39/1
  Bus Creator5/1 -> HRInput/1
  MC_HR_DataTag/1 -> Data Type Conversion37/1
  Data Type Conversion36/1 -> Bus Creator5/1

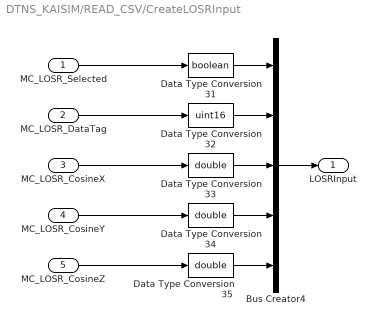
== system DTNS_KAISIM/READ_CSV/CreateLOSRInput ==
  MC_LOSR_Selected : Inport
  MC_LOSR_DataTag : Inport  Port=2
  MC_LOSR_CosineX : Inport  Port=3
  MC_LOSR_CosineY : Inport  Port=4
  MC_LOSR_CosineZ : Inport  Port=5
  Bus Creator4 : BusCreator  Inputs=5  OutDataTypeStr=Bus: LOSRInput  NonVirtualBus=on
      settings: InheritFromInputs=off
  Data Type Conversion31 : DataTypeConversion  OutDataTypeStr=boolean  RndMeth=Nearest  SaturateOnIntegerOverflow=off
  Data Type Conversion32 : DataTypeConversion  OutDataTypeStr=uint16  RndMeth=Nearest  SaturateOnIntegerOverflow=off
  Data Type Conversion33 : DataTypeConversion  OutDataTypeStr=double  RndMeth=Nearest  SaturateOnIntegerOverflow=off
  Data Type Conversion34 : DataTypeConversion  OutDataTypeStr=double  RndMeth=Nearest  SaturateOnIntegerOverflow=off
  Data Type Conversion35 : DataTypeConversion  OutDataTypeStr=double  RndMeth=Nearest  SaturateOnIntegerOverflow=off
  LOSRInput : Outport
  wires:
  MC_LOSR_Selected/1 -> Data Type Conversion31/1
  MC_LOSR_DataTag/1 -> Data Type Conversion32/1
  Data Type Conversion34/1 -> Bus Creator4/4
  Data Type Conversion33/1 -> Bus Creator4/3
  MC_LOSR_CosineZ/1 -> Data Type Conversion35/1
  MC_LOSR_CosineX/1 -> Data Type Conversion33/1
  Data Type Conversion31/1 -> Bus Creator4/1
  Data Type Conversion35/1 -> Bus Creator4/5
  Data Type Conversion32/1 -> Bus Creator4/2
  MC_LOSR_CosineY/1 -> Data Type Conversion34/1
  Bus Creator4/1 -> LOSRInput/1

== system DTNS_KAISIM/READ_CSV/CreateTRNInput ==
  INS_In : Inport  OutDataTypeStr=Bus: TRN_INS
  GPS_In : Inport  Port=2  OutDataTypeStr=Bus: TRN_GPS
  RALT_In : Inport  Port=3  OutDataTypeStr=Bus: TRN_RALT
  MC_In : Inport  Port=4  OutDataTypeStr=Bus: TRN_MC
  Dataprocess1 : Subsystem
  TRN INPUT : Outport  OutDataTypeStr=Bus: TRNInput  VectorParamsAs1DForOutWhenUnconnected=off
  wires:
  GPS_In/1 -> Dataprocess1/1(In_GPS)
  Dataprocess1/1(TRN INPUT) -> TRN INPUT/1
  RALT_In/1 -> Dataprocess1/3(In_RALT)
  MC_In/1 -> Dataprocess1/4(IN_MC)
  INS_In/1 -> Dataprocess1/2(In_INS)

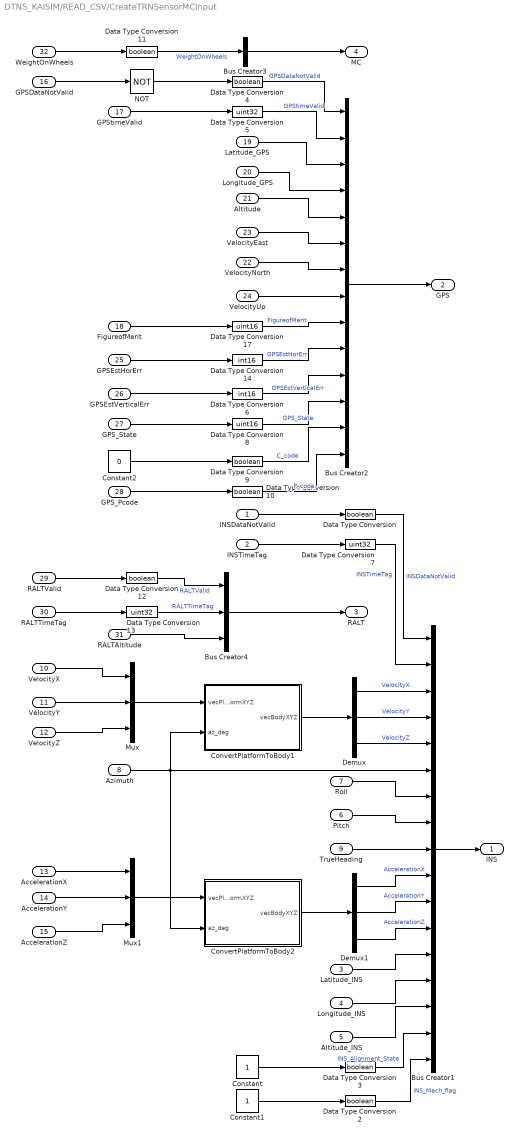
== system DTNS_KAISIM/READ_CSV/CreateTRNSensorMCInput ==
  INSDataNotValid : Inport
  INSTimeTag : Inport  Port=2
  Latitude_INS : Inport  Port=3
  Longitude_INS : Inport  Port=4
  Altitude_INS : Inport  Port=5
  Pitch : Inport  Port=6
  Roll : Inport  Port=7
  Azimuth : Inport  Port=8
  TrueHeading : Inport  Port=9
  VelocityX : Inport  Port=10
  VelocityY : Inport  Port=11
  VelocityZ : Inport  Port=12
  AccelerationX : Inport  Port=13
  AccelerationY : Inport  Port=14
  AccelerationZ : Inport  Port=15
  GPSDataNotValid : Inport  Port=16
  GPStimeValid : Inport  Port=17
  FigureofMerit : Inport  Port=18
  Latitude_GPS : Inport  Port=19
  Longitude_GPS : Inport  Port=20
  Altitude : Inport  Port=21
  VelocityNorth : Inport  Port=22
  VelocityEast : Inport  Port=23
  VelocityUp : Inport  Port=24
  GPSEstHorErr : Inport  Port=25
  GPSEstVerticalErr : Inport  Port=26
  GPS_State : Inport  Port=27
  GPS_Pcode : Inport  Port=28
  RALTValid : Inport  Port=29
  RALTTimeTag : Inport  Port=30
  RALTAltitude : Inport  Port=31
  WeightOnWheels : Inport  Port=32
  Bus Creator1 : BusCreator  Inputs=17  OutDataTypeStr=Bus: TRN_INS  NonVirtualBus=on
      settings: InheritFromInputs=off
  Bus Creator2 : BusCreator  Inputs=14  OutDataTypeStr=Bus: TRN_GPS  NonVirtualBus=on
      settings: InheritFromInputs=off
  Bus Creator3 : BusCreator  Inputs=1  OutDataTypeStr=Bus: TRN_MC  NonVirtualBus=on
      settings: InheritFromInputs=off
  Bus Creator4 : BusCreator  Inputs=3  OutDataTypeStr=Bus: TRN_RALT  NonVirtualBus=on
      settings: InheritFromInputs=off
  Constant : Constant
  Constant1 : Constant
  Constant2 : Constant  Value=0
  ConvertPlatformToBody1 : MATLAB Function  TreatAsAtomicUnit=on
  ConvertPlatformToBody2 : MATLAB Function  TreatAsAtomicUnit=on
  Data Type Conversion{,2..4,9..12} (8 alike) : DataTypeConversion  OutDataTypeStr=boolean  SaturateOnIntegerOverflow=off  RndMeth=Floor
  Data Type Conversion13 : DataTypeConversion  OutDataTypeStr=uint32  SaturateOnIntegerOverflow=off  RndMeth=Floor
  Data Type Conversion14 : DataTypeConversion  OutDataTypeStr=int16  SaturateOnIntegerOverflow=off  RndMeth=Floor
  Data Type Conversion17 : DataTypeConversion  OutDataTypeStr=uint16  SaturateOnIntegerOverflow=off  RndMeth=Floor
  Data Type Conversion5 : DataTypeConversion  OutDataTypeStr=uint32  SaturateOnIntegerOverflow=off  RndMeth=Floor
  Data Type Conversion6 : DataTypeConversion  OutDataTypeStr=int16  SaturateOnIntegerOverflow=off  RndMeth=Floor
  Data Type Conversion7 : DataTypeConversion  OutDataTypeStr=uint32  SaturateOnIntegerOverflow=off  RndMeth=Floor
  Data Type Conversion8 : DataTypeConversion  OutDataTypeStr=uint16  SaturateOnIntegerOverflow=off  RndMeth=Floor
  Demux : Demux  Outputs=3
  Demux1 : Demux  Outputs=3
  Mux : Mux  Inputs=3
  Mux1 : Mux  Inputs=3
  NOT : Logic  Operator=NOT  IconShape=distinctive  AllPortsSameDT=off  OutDataTypeStr=boolean
  INS : Outport
  GPS : Outport  Port=2
  RALT : Outport  Port=3
  MC : Outport  Port=4
  wires:
  RALTValid/1 -> Data Type Conversion12/1
  RALTTimeTag/1 -> Data Type Conversion13/1
  GPS_Pcode/1 -> Data Type Conversion10/1
  RALTAltitude/1 -> Bus Creator4/3
  Mux1/1 -> ConvertPlatformToBody2/1(vecPlatformXYZ)
  ConvertPlatformToBody2/1(vecBodyXYZ) -> Demux1/1
  AccelerationY/1 -> Mux1/2
  VelocityZ/1 -> Mux/3
  AccelerationX/1 -> Mux1/1
  AccelerationZ/1 -> Mux1/3
  ConvertPlatformToBody1/1(vecBodyXYZ) -> Demux/1
  Mux/1 -> ConvertPlatformToBody1/1(vecPlatformXYZ)
  VelocityX/1 -> Mux/1
  TrueHeading/1 -> Bus Creator1/9
  VelocityY/1 -> Mux/2
  Bus Creator4/1 -> RALT/1
  Longitude_INS/1 -> Bus Creator1/14
  Pitch/1 -> Bus Creator1/8
  Altitude_INS/1 -> Bus Creator1/15
  Roll/1 -> Bus Creator1/7
  GPS_State/1 -> Data Type Conversion8/1
  GPSEstHorErr/1 -> Data Type Conversion14/1
  GPSEstVerticalErr/1 -> Data Type Conversion6/1
  VelocityUp/1 -> Bus Creator2/8
  Latitude_GPS/1 -> Bus Creator2/3
  GPSDataNotValid/1 -> NOT/1
  FigureofMerit/1 -> Data Type Conversion17/1
  GPStimeValid/1 -> Data Type Conversion5/1
  VelocityEast/1 -> Bus Creator2/6
  Altitude/1 -> Bus Creator2/5
  VelocityNorth/1 -> Bus Creator2/7
  Longitude_GPS/1 -> Bus Creator2/4
  Latitude_INS/1 -> Bus Creator1/13
  INSDataNotValid/1 -> Data Type Conversion/1
  INSTimeTag/1 -> Data Type Conversion7/1
  Bus Creator2/1 -> GPS/1
  Bus Creator3/1 -> MC/1
  Demux1/1 -> Bus Creator1/10  "AccelerationX"
  Demux1/2 -> Bus Creator1/11  "AccelerationY"
  Demux1/3 -> Bus Creator1/12  "AccelerationZ"
  Demux/3 -> Bus Creator1/5  "VelocityZ"
  Demux/1 -> Bus Creator1/3  "VelocityX"
  Demux/2 -> Bus Creator1/4  "VelocityY"
  Constant/1 -> Data Type Conversion3/1
  Constant2/1 -> Data Type Conversion9/1
  Constant1/1 -> Data Type Conversion2/1
  Bus Creator1/1 -> INS/1
  Data Type Conversion10/1 -> Bus Creator2/14  "P_code"
  Data Type Conversion11/1 -> Bus Creator3/1  "WeightOnWheels"
  WeightOnWheels/1 -> Data Type Conversion11/1
  Data Type Conversion7/1 -> Bus Creator1/2  "INSTimeTag"
  Data Type Conversion6/1 -> Bus Creator2/11  "GPSEstVerticalErr"
  NOT/1 -> Data Type Conversion4/1
  Data Type Conversion12/1 -> Bus Creator4/1  "RALTValid"
  Data Type Conversion13/1 -> Bus Creator4/2  "RALTTimeTag"
  Data Type Conversion9/1 -> Bus Creator2/13  "C_code"
  Data Type Conversion8/1 -> Bus Creator2/12  "GPS_State"
  Data Type Conversion14/1 -> Bus Creator2/10  "GPSEstHorErr"
  Data Type Conversion17/1 -> Bus Creator2/9  "FigureofMerit"
  Data Type Conversion4/1 -> Bus Creator2/1  "GPSDataNotValid"
  Data Type Conversion5/1 -> Bus Creator2/2  "GPStimeValid"
  Data Type Conversion2/1 -> Bus Creator1/17  "INS_Mech_flag"
  Data Type Conversion3/1 -> Bus Creator1/16  "INS_Alignment_State"
  Data Type Conversion/1 -> Bus Creator1/1  "INSDataNotValid"
  Azimuth/1 -> ConvertPlatformToBody2/2(az_deg), ConvertPlatformToBody1/2(az_deg), Bus Creator1/6

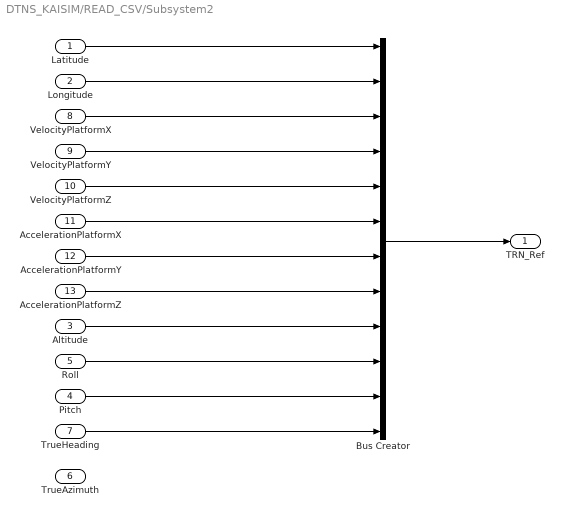
== system DTNS_KAISIM/READ_CSV/Subsystem2 ==
  Latitude : Inport
  Longitude : Inport  Port=2
  Altitude : Inport  Port=3
  Pitch : Inport  Port=4
  Roll : Inport  Port=5
  TrueAzimuth : Inport  Port=6
  TrueHeading : Inport  Port=7
  VelocityPlatformX : Inport  Port=8
  VelocityPlatformY : Inport  Port=9
  VelocityPlatformZ : Inport  Port=10
  AccelerationPlatformX : Inport  Port=11
  AccelerationPlatformY : Inport  Port=12
  AccelerationPlatformZ : Inport  Port=13
  Bus Creator : BusCreator  Inputs=12  OutDataTypeStr=Bus: TRN_Ref  NonVirtualBus=on
      settings: InheritFromInputs=off
  TRN_Ref : Outport
  wires:
  Bus Creator/1 -> TRN_Ref/1
  Latitude/1 -> Bus Creator/1
  Longitude/1 -> Bus Creator/2
  VelocityPlatformX/1 -> Bus Creator/3
  VelocityPlatformY/1 -> Bus Creator/4
  VelocityPlatformZ/1 -> Bus Creator/5
  AccelerationPlatformX/1 -> Bus Creator/6
  AccelerationPlatformY/1 -> Bus Creator/7
  AccelerationPlatformZ/1 -> Bus Creator/8
  Altitude/1 -> Bus Creator/9
  Roll/1 -> Bus Creator/10
  Pitch/1 -> Bus Creator/11
  TrueHeading/1 -> Bus Creator/12

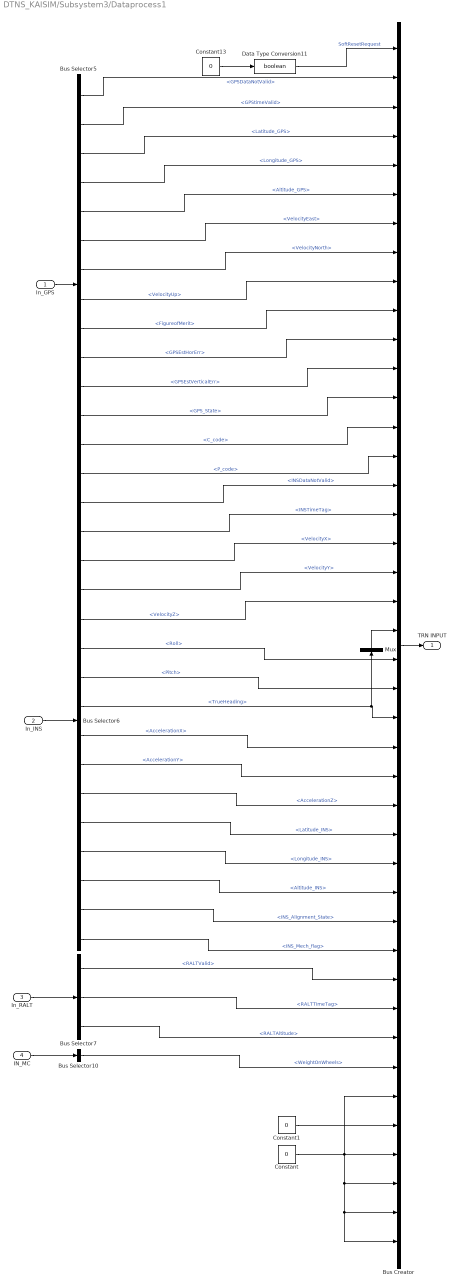
== system DTNS_KAISIM/Subsystem3/Dataprocess1 ==
  In_GPS : Inport
  In_INS : Inport  Port=2
  In_RALT : Inport  Port=3
  IN_MC : Inport  Port=4
  Bus Creator : BusCreator  Inputs=42  OutDataTypeStr=Bus: TRNInput
      settings: InheritFromInputs=off
  Bus Selector10 : BusSelector  OutputSignals=WeightOnWheels
  Bus Selector5 : BusSelector  OutputSignals=GPSDataNotValid,GPStimeValid,Latitude_GPS,Longitude_GPS,Altitude_GPS,VelocityEast,VelocityNorth,VelocityUp,FigureofMerit,GPSEstHorErr,GPSEstVerticalErr,GPS_State,C_code,P_code
  Bus Selector6 : BusSelector  OutputSignals=INSDataNotValid,INSTimeTag,VelocityX,VelocityY,VelocityZ,Roll,Pitch,TrueHeading,AccelerationX,AccelerationY,AccelerationZ,Latitude_INS,Longitude_INS,Altitude_INS,INS_Alignment_State,INS_Mech_flag
  Bus Selector7 : BusSelector  OutputSignals=RALTValid,RALTTimeTag,RALTAltitude
  Constant : Constant  Value=0
  Constant1 : Constant  Value=0  OutDataTypeStr=uint32
  Constant13 : Constant  Value=0
  Data Type Conversion11 : DataTypeConversion  OutDataTypeStr=boolean  SaturateOnIntegerOverflow=off  RndMeth=Floor
  Mux : Mux  Inputs=1
  TRN INPUT : Outport  OutDataTypeStr=Bus: TRNInput  VectorParamsAs1DForOutWhenUnconnected=off
  wires:
  IN_MC/1 -> Bus Selector10/1
  In_RALT/1 -> Bus Selector7/1
  Constant13/1 -> Data Type Conversion11/1
  In_INS/1 -> Bus Selector6/1
  Data Type Conversion11/1 -> Bus Creator/1  "SoftResetRequest"
  In_GPS/1 -> Bus Selector5/1
  Bus Selector5/2 -> Bus Creator/3  "<GPStimeValid>"
  Bus Selector5/5 -> Bus Creator/6  "<Altitude_GPS>"
  Bus Selector5/6 -> Bus Creator/7  "<VelocityEast>"
  Bus Selector5/7 -> Bus Creator/8  "<VelocityNorth>"
  Bus Selector5/8 -> Bus Creator/9  "<VelocityUp>"
  Bus Selector5/9 -> Bus Creator/10  "<FigureofMerit>"
  Bus Selector5/10 -> Bus Creator/11  "<GPSEstHorErr>"
  Bus Selector5/11 -> Bus Creator/12  "<GPSEstVerticalErr>"
  Bus Selector5/12 -> Bus Creator/13  "<GPS_State>"
  Bus Selector5/13 -> Bus Creator/14  "<C_code>"
  Bus Selector5/14 -> Bus Creator/15  "<P_code>"
  Bus Selector6/1 -> Bus Creator/16  "<INSDataNotValid>"
  Bus Selector6/2 -> Bus Creator/17  "<INSTimeTag>"
  Bus Selector6/3 -> Bus Creator/18  "<VelocityX>"
  Bus Selector6/4 -> Bus Creator/19  "<VelocityY>"
  Bus Selector6/5 -> Bus Creator/20  "<VelocityZ>"
  Bus Selector5/4 -> Bus Creator/5  "<Longitude_GPS>"
  Bus Selector5/3 -> Bus Creator/4  "<Latitude_GPS>"
  Bus Selector5/1 -> Bus Creator/2  "<GPSDataNotValid>"
  Constant/1 -> Bus Creator/37, Bus Creator/39, Bus Creator/40, Bus Creator/41, Bus Creator/42
  Constant1/1 -> Bus Creator/38
  Bus Selector6/6 -> Bus Creator/22  "<Roll>"
  Bus Selector6/7 -> Bus Creator/23  "<Pitch>"
  Bus Selector6/8 -> Bus Creator/24, Mux/1  "<TrueHeading>"
  Bus Selector6/9 -> Bus Creator/25  "<AccelerationX>"
  Bus Selector6/10 -> Bus Creator/26  "<AccelerationY>"
  Bus Selector6/11 -> Bus Creator/27  "<AccelerationZ>"
  Bus Selector6/12 -> Bus Creator/28  "<Latitude_INS>"
  Bus Selector6/13 -> Bus Creator/29  "<Longitude_INS>"
  Bus Selector6/14 -> Bus Creator/30  "<Altitude_INS>"
  Bus Selector6/15 -> Bus Creator/31  "<INS_Alignment_State>"
  Bus Selector6/16 -> Bus Creator/32  "<INS_Mech_flag>"
  Bus Selector7/1 -> Bus Creator/33  "<RALTValid>"
  Bus Selector7/2 -> Bus Creator/34  "<RALTTimeTag>"
  Bus Selector7/3 -> Bus Creator/35  "<RALTAltitude>"
  Bus Selector10/1 -> Bus Creator/36  "<WeightOnWheels>"
  Bus Creator/1 -> TRN INPUT/1
  Mux/1 -> Bus Creator/21

== system DTNS_KAISIM/LogData_process/InitUpdateMapCache/Caching ==
  lat : Inport
  lon : Inport  Port=2
  Action Port : ActionPort
  FTGMapCaching1 : MATLAB Function  TreatAsAtomicUnit=on
  Scope : Scope  NumInputPorts=3
  wires:
  lat/1 -> FTGMapCaching1/1(lat), Scope/1
  lon/1 -> FTGMapCaching1/2(lon), Scope/2
  FTGMapCaching1/3(hDEM) -> Scope/3

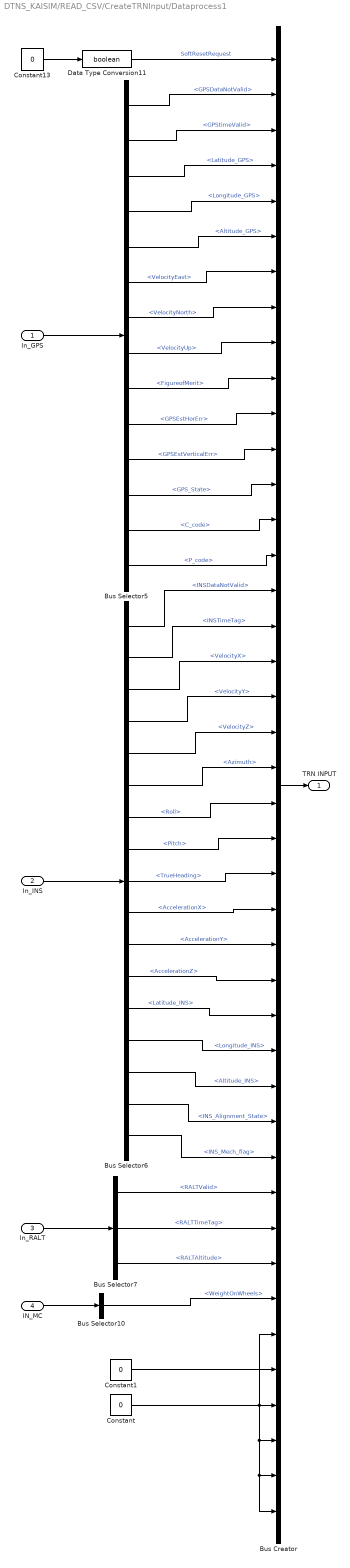
== system DTNS_KAISIM/READ_CSV/CreateTRNInput/Dataprocess1 ==
  In_GPS : Inport
  In_INS : Inport  Port=2
  In_RALT : Inport  Port=3
  IN_MC : Inport  Port=4
  Bus Creator : BusCreator  Inputs=42  OutDataTypeStr=Bus: TRNInput
      settings: InheritFromInputs=off
  Bus Selector10 : BusSelector  OutputSignals=WeightOnWheels
  Bus Selector5 : BusSelector  OutputSignals=GPSDataNotValid,GPStimeValid,Latitude_GPS,Longitude_GPS,Altitude_GPS,VelocityEast,VelocityNorth,VelocityUp,FigureofMerit,GPSEstHorErr,GPSEstVerticalErr,GPS_State,C_code,P_code
  Bus Selector6 : BusSelector  OutputSignals=INSDataNotValid,INSTimeTag,VelocityX,VelocityY,VelocityZ,Azimuth,Roll,Pitch,TrueHeading,AccelerationX,AccelerationY,AccelerationZ,Latitude_INS,Longitude_INS,Altitude_INS,INS_Alignment_State,INS_Mech_flag
  Bus Selector7 : BusSelector  OutputSignals=RALTValid,RALTTimeTag,RALTAltitude
  Constant : Constant  Value=0
  Constant1 : Constant  Value=0  OutDataTypeStr=uint32
  Constant13 : Constant  Value=0
  Data Type Conversion11 : DataTypeConversion  OutDataTypeStr=boolean  SaturateOnIntegerOverflow=off  RndMeth=Floor
  TRN INPUT : Outport  OutDataTypeStr=Bus: TRNInput  VectorParamsAs1DForOutWhenUnconnected=off
  wires:
  Bus Selector6/4 -> Bus Creator/19  "<VelocityY>"
  Bus Selector6/5 -> Bus Creator/20  "<VelocityZ>"
  Bus Selector6/7 -> Bus Creator/22  "<Roll>"
  Bus Selector6/6 -> Bus Creator/21  "<Azimuth>"
  Bus Creator/1 -> TRN INPUT/1
  Bus Selector7/2 -> Bus Creator/34  "<RALTTimeTag>"
  Bus Selector7/1 -> Bus Creator/33  "<RALTValid>"
  Bus Selector6/16 -> Bus Creator/31  "<INS_Alignment_State>"
  Bus Selector5/2 -> Bus Creator/3  "<GPStimeValid>"
  Bus Selector5/1 -> Bus Creator/2  "<GPSDataNotValid>"
  Bus Selector10/1 -> Bus Creator/36  "<WeightOnWheels>"
  Constant/1 -> Bus Creator/41, Bus Creator/42, Bus Creator/40, Bus Creator/37, Bus Creator/39
  Constant13/1 -> Data Type Conversion11/1
  Constant1/1 -> Bus Creator/38
  Bus Selector7/3 -> Bus Creator/35  "<RALTAltitude>"
  Bus Selector6/17 -> Bus Creator/32  "<INS_Mech_flag>"
  Bus Selector6/12 -> Bus Creator/27  "<AccelerationZ>"
  Bus Selector6/13 -> Bus Creator/28  "<Latitude_INS>"
  Bus Selector6/14 -> Bus Creator/29  "<Longitude_INS>"
  Bus Selector6/15 -> Bus Creator/30  "<Altitude_INS>"
  Bus Selector6/8 -> Bus Creator/23  "<Pitch>"
  Bus Selector6/9 -> Bus Creator/24  "<TrueHeading>"
  Bus Selector6/10 -> Bus Creator/25  "<AccelerationX>"
  Bus Selector6/11 -> Bus Creator/26  "<AccelerationY>"
  Bus Selector5/5 -> Bus Creator/6  "<Altitude_GPS>"
  Bus Selector5/6 -> Bus Creator/7  "<VelocityEast>"
  Bus Selector5/4 -> Bus Creator/5  "<Longitude_GPS>"
  Bus Selector5/3 -> Bus Creator/4  "<Latitude_GPS>"
  Bus Selector6/1 -> Bus Creator/16  "<INSDataNotValid>"
  Bus Selector6/2 -> Bus Creator/17  "<INSTimeTag>"
  Bus Selector6/3 -> Bus Creator/18  "<VelocityX>"
  Bus Selector5/11 -> Bus Creator/12  "<GPSEstVerticalErr>"
  Bus Selector5/12 -> Bus Creator/13  "<GPS_State>"
  Bus Selector5/13 -> Bus Creator/14  "<C_code>"
  Bus Selector5/14 -> Bus Creator/15  "<P_code>"
  Bus Selector5/7 -> Bus Creator/8  "<VelocityNorth>"
  Bus Selector5/8 -> Bus Creator/9  "<VelocityUp>"
  Bus Selector5/9 -> Bus Creator/10  "<FigureofMerit>"
  Bus Selector5/10 -> Bus Creator/11  "<GPSEstHorErr>"
  IN_MC/1 -> Bus Selector10/1
  In_RALT/1 -> Bus Selector7/1
  In_INS/1 -> Bus Selector6/1
  In_GPS/1 -> Bus Selector5/1
  Data Type Conversion11/1 -> Bus Creator/1  "SoftResetRequest"
